simulink model "coprim"  (R2021b)
settings: Solver=VariableStepAuto  StartTime=0.0  StopTime=10.0  RelTol=1e-3
undefined symbols (not defined in the file): A, B, BB, C, D, DD, L, sigma_ay, sigma_r
libraries: simulink x2
settings Model: Creator=Sazgar  LastModifiedBy=Sazgar

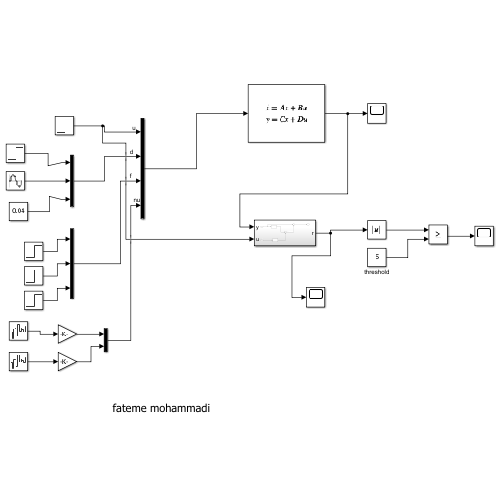
[thumbnail: Simulink's stored preview of the top-level diagram]
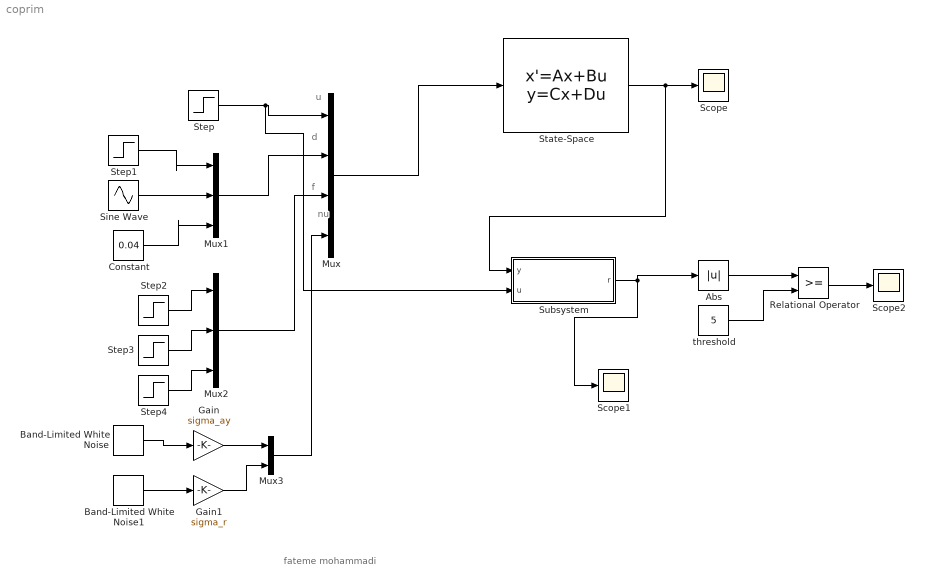
== system coprim ==
  note: fateme mohammadi
  note: f
  note: nu
  note: d
  note: u
  Abs : Abs
  Band-Limited White Noise : simulink/Sources/Band-Limited White Noise  Cov=[1]  Ts=0.01  seed=[1234]
  Band-Limited White Noise1 : simulink/Sources/Band-Limited White Noise  Cov=[1]  Ts=0.01  seed=[5678]
  Constant : Constant  Value=0.04  SampleTime=0.01
  Gain : Gain  Gain=sigma_ay
  Gain1 : Gain  Gain=sigma_r
  Mux : Mux
  Mux1 : Mux  Inputs=3
  Mux2 : Mux  Inputs=3
  Mux3 : Mux  Inputs=2
  Relational Operator : RelationalOperator  OutDataTypeStr=boolean  RndMeth=Simplest
  Scope : Scope
  Scope1 : Scope
  Scope2 : Scope
  Sine Wave : Sin  Amplitude=0.03  Frequency=0.5  SampleTime=0.01
  State-Space : StateSpace  A=A  B=BB  C=C  D=DD  InitialCondition=0
  Step : Step  SampleTime=0.01
  Step1 : Step  Time=3  After=0.05  SampleTime=0.01
  Step2 : Step  Time=3  SampleTime=0.01
  Step3 : Step  Time=5  After=0.5  SampleTime=0.01
  Step4 : Step  Time=7  After=0.8  SampleTime=0.01
  Subsystem : Subsystem
  threshold : Constant  Value=5
  wires:
  Step4/1 -> Mux2/3
  Mux1/1 -> Mux/2
  Band-Limited White Noise1/1 -> Gain1/1
  Band-Limited White Noise/1 -> Gain/1
  Gain/1 -> Mux3/1
  Gain1/1 -> Mux3/2
  Step2/1 -> Mux2/1
  Constant/1 -> Mux1/3
  Step/1 -> Subsystem/2(u), Mux/1
  Sine Wave/1 -> Mux1/2
  Step3/1 -> Mux2/2
  Step1/1 -> Mux1/1
  Mux2/1 -> Mux/3
  Mux3/1 -> Mux/4
  Mux/1 -> State-Space/1
  State-Space/1 -> Subsystem/1(y), Scope/1
  Subsystem/1(r) -> Scope1/1, Abs/1
  threshold/1 -> Relational Operator/2
  Abs/1 -> Relational Operator/1
  Relational Operator/1 -> Scope2/1

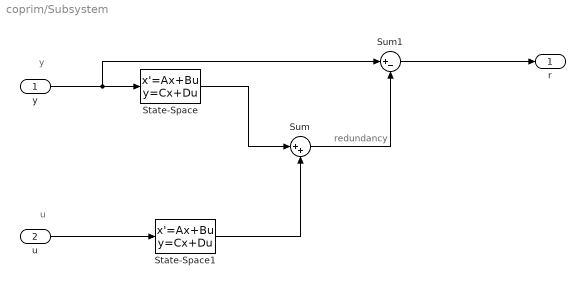
== system coprim/Subsystem ==
  note: redundancy
  note: u
  note: y
  y : Inport
  u : Inport  Port=2
  State-Space : StateSpace  A=A-L*C  B=L  C=C  D=zeros(2)  InitialCondition=0
  State-Space1 : StateSpace  A=A-L*C  B=B-L*D  C=C  D=D  InitialCondition=0
  Sum : Sum  Inputs=|++
  Sum1 : Sum  Inputs=|+-
  r : Outport
  wires:
  u/1 -> State-Space1/1
  y/1 -> Sum1/1, State-Space/1
  State-Space/1 -> Sum/1
  State-Space1/1 -> Sum/2
  Sum/1 -> Sum1/2
  Sum1/1 -> r/1
